simulink model "mathModel2"  (R2021a)
settings: Solver=VariableStepAuto  StartTime=0.0  StopTime=inf  RelTol=1e-3
libraries: slrealtimeutilitieslib x2, slrealtimeiplib x2, sldrtlib x1
settings Model: Creator=proku  LastModifiedBy=proku
settings DebuggingCC: SignalInfNanChecking=error

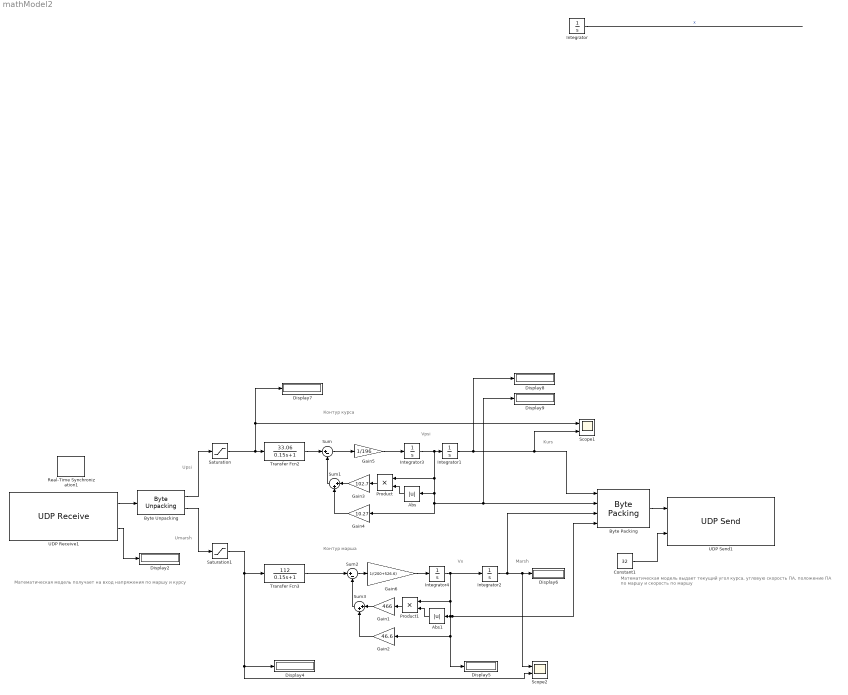
== system mathModel2 ==
  note: Математическая модель получает на вход
      | напряжения по маршу и курсу
  note: Marsh
  note: Vx
  note: Kurs
  note: Umarsh
  note: Upsi
  note: Vpsi
  note: Математическая модель выдает текущий угол курса, угловую скорость ПА, положение ПА по маршу и скорость по маршу
  note: Контур курса
  note: Контур марша
  Abs : Abs
  Abs1 : Abs
  "Byte Packing " : slrealtimeutilitieslib/Byte Packing  MaskPackedDataType=uint8  MaskUnpackedDataTypes={'double','double','double','double'}  MaskAlignment=1
  "Byte Unpacking " : slrealtimeutilitieslib/Byte Unpacking  MaskUnpackedDataTypes={'double','double'}  MaskUnpackedDataSizes={[1],[1]}  MaskAlignment=1
      settings: SourceProductBaseCode=XP
  Constant1 : Constant  Value=32
  Display{2,4..9} (7 alike) : Display
  Gain1 : Gain  Gain=466
  Gain2 : Gain  Gain=46.6
  Gain3 : Gain  Gain=102.7
  Gain4 : Gain  Gain=10.27
  Gain5 : Gain  Gain=1/196
  Gain6 : Gain  Gain=1/(200+526.6)
  Integrator{,1..4} (5 alike) : Integrator
  Product : Product
  Product1 : Product
  Real-Time Synchronization1 : sldrtlib/Real-Time Synchronization  SampleTime=0.01  MaxMissedTicks=10000  ShowMissedTicks=on  YieldWhenWaiting=off
  Saturation : Saturate  UpperLimit=12  LowerLimit=-12
  Saturation1 : Saturate  UpperLimit=12  LowerLimit=-12
  Scope1 : Scope  NumInputPorts=2
  Scope2 : Scope  NumInputPorts=2
  Sum : Sum  Inputs=|+-
  Sum1 : Sum  Inputs=|++
  Sum2 : Sum  Inputs=|+-
  Sum3 : Sum  Inputs=|++
  Transfer Fcn2 : TransferFcn  Numerator=[33.06]  Denominator=[0.15 1]
  Transfer Fcn3 : TransferFcn  Numerator=[112]  Denominator=[0.15 1]
  UDP Receive1 : slrealtimeiplib/UDP Receive  useHostTargetConn=on  ipAddress=10.10.10.15  localPort=13042  rcvWidth=16  rcvFmAny=on  fmAddress=0.0.0.0  sampleTime=0.01
      settings: SourceProductBaseCode=XP
  UDP Send1 : slrealtimeiplib/UDP Send  useHostTargetConn=on  ipAddress=10.10.10.15  localPort=13043  toAddress=127.0.0.1  toPort=13044  sampleTime=0.01
      settings: SourceProductBaseCode=XP
  wires:
  UDP Receive1/2 -> Display2/1
  Product1/1 -> Gain1/1
  Integrator1/1 -> Scope1/2, "Byte Packing "/1, Display8/1
  Gain3/1 -> Sum1/1
  Sum/1 -> Gain5/1
  Gain2/1 -> Sum3/2
  Gain4/1 -> Sum1/2
  Gain1/1 -> Sum3/1
  Gain5/1 -> Integrator3/1
  "Byte Packing "/1 -> UDP Send1/1
  Abs1/1 -> Product1/2
  Constant1/1 -> UDP Send1/2
  Transfer Fcn3/1 -> Sum2/1
  UDP Receive1/1 -> "Byte Unpacking "/1
  Sum2/1 -> Gain6/1
  Integrator4/1 -> "Byte Packing "/4, Abs1/1, Gain2/1, Display5/1, Product1/1, Integrator2/1
  Abs/1 -> Product/2
  Integrator3/1 -> "Byte Packing "/2, Display9/1, Gain4/1, Abs/1, Product/1, Integrator1/1
  Transfer Fcn2/1 -> Sum/1
  Sum3/1 -> Sum2/2
  Product/1 -> Gain3/1
  Gain6/1 -> Integrator4/1
  Sum1/1 -> Sum/2
  Integrator2/1 -> Scope2/1, Display6/1, "Byte Packing "/3
  "Byte Unpacking "/1 -> Saturation/1
  "Byte Unpacking "/2 -> Saturation1/1
  Integrator/1 -> ?  "x"
  Saturation/1 -> Display7/1, Scope1/1, Transfer Fcn2/1
  Saturation1/1 -> Scope2/2, Display4/1, Transfer Fcn3/1
